simulink model "Desain_AMC"  (R2023a)
settings: Solver=VariableStepAuto  StartTime=0.0  StopTime=0.5  RelTol=1e-3
libraries: spsSeriesRLCBranchLib x18, dspstat3 x11, spsVoltageMeasurementLib x8, spsCurrentMeasurementLib x4, eePowerMeasurement x4, spsACVoltageSourceLib x2, spsDCVoltageSourceLib x2, spsRMSLib x1, sps_lib x1
settings Model: Creator=rne2p  LastModifiedBy=rne2p

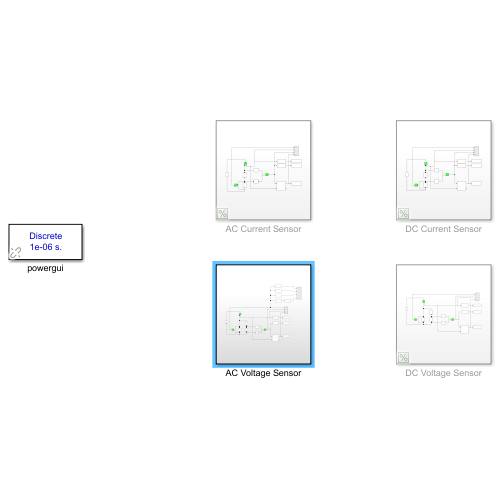
[thumbnail: Simulink's stored preview of the top-level diagram]
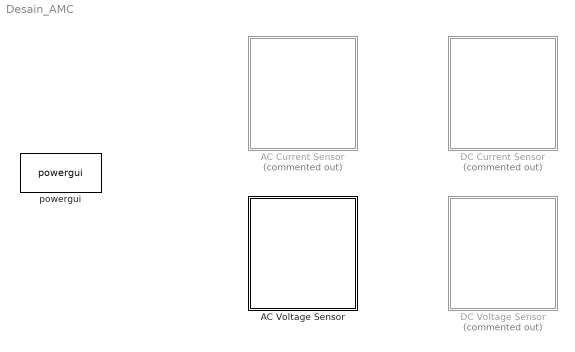
== system Desain_AMC ==
  AC Current Sensor : Subsystem  Commented=on
  AC Voltage Sensor : Subsystem
  DC Current Sensor : Subsystem  Commented=on
  DC Voltage Sensor : Subsystem  Commented=on
  powergui : sps_lib/powergui  Priority=1  SimulationMode=Discrete  SampleTime=1e-6  frequency=60  Iterations=50  frequencyindice=50  Pbase=100e6  ErrMax=1e-4  UnitsV=kV  UnitsW=MW  buscounter=0  FunctionMessages=off  echomessages=off  EnableUseOfTLC=off  CurrentSourceSwitches=off  DisableSnubberDevices=off  DisableRonSwitches=off  DisableVfSwitches=off  DisplayEquations=off  AutomaticDiscreteSolvers=off  SolverType=Tustin/Backward Euler (TBE)  Interpol=off  ExternalGateDelay=off  methode=off  Ts=100  x0status=blocks  SPID=on  SwTol=0  HookPort=off  NonlinearTolerance=1e-4  nMaxIteration=100  ContinueOnMaxIteration=off  RestoreLinks=warning  ResistiveCurrentMeasurement=off  Frange=[0:2:500]  Ylog=off  Xlog=on  ShowGrid=off  save=off  variable=ZData  structure=0  ZoomFFT=off  StartTime=0.0  cycles=1  DisplayStyle=1  fundamental=60  FreqAxis=off  MaxFrequency=1000  frequencyindicesteady=1  RmsSteady=1  display=off

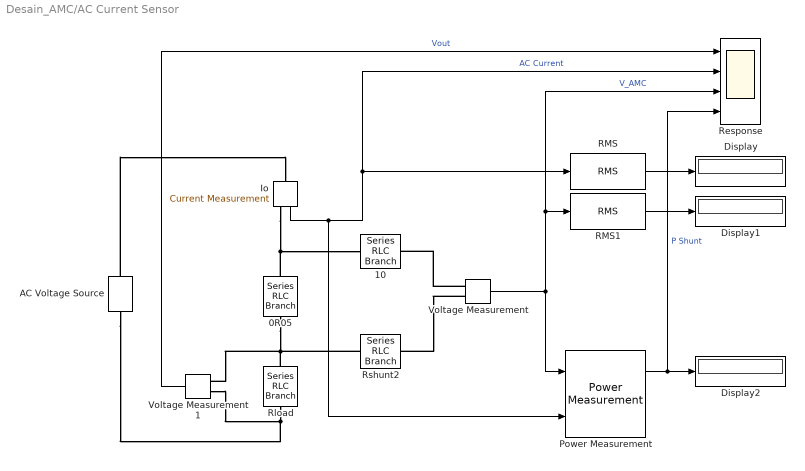
== system Desain_AMC/AC Current Sensor ==
  0R05 : spsSeriesRLCBranchLib/Series RLC Branch  LConnTagsString=__new0  RConnTagsString=__new0  BranchType=R  Resistance=50e-3  Inductance=100e-03  SetiL0=off  InitialCurrent=0  Capacitance=1.0  Setx0=off  InitialVoltage=0  Measurements=None
  10 : spsSeriesRLCBranchLib/Series RLC Branch  LConnTagsString=__new0  RConnTagsString=__new0  BranchType=R  Resistance=100  Inductance=100e-03  SetiL0=off  InitialCurrent=0  Capacitance=1.0  Setx0=off  InitialVoltage=0  Measurements=None
  AC Voltage Source : spsACVoltageSourceLib/AC Voltage Source  Amplitude=220*sqrt(2)  Phase=0  Frequency=50  SampleTime=0  Measurements=None  BusType=swing  Pref=10e3  Qref=0  Qmin=-inf  Qmax=+inf
  Display : Display
  Display1 : Display
  Display2 : Display
  Io : spsCurrentMeasurementLib/Current Measurement  Tag=PoWeRsYsTeMmEaSuReMeNt  PhasorSimulation=off  OutputType=Magnitude  PSBequivalent=0
      settings: AttributesFormatString=\n
  Power Measurement : eePowerMeasurement/Power Measurement  LabelModeActiveChoice=Continuous  F=50  K=1  Ts=0
  RMS : dspstat3/RMS  run=on  directionMode=Each column  dimension=1  InputProcessing=Columns as channels (frame based)  reset_popup=None
  RMS1 : dspstat3/RMS  run=on  directionMode=Each column  dimension=1  InputProcessing=Columns as channels (frame based)  reset_popup=None
  Response : Scope  NumInputPorts=4
  Rload : spsSeriesRLCBranchLib/Series RLC Branch  LConnTagsString=__new0  RConnTagsString=__new0  BranchType=R  Resistance=220/1  Inductance=100e-03  SetiL0=off  InitialCurrent=0  Capacitance=1.0  Setx0=off  InitialVoltage=0  Measurements=None
  Rshunt2 : spsSeriesRLCBranchLib/Series RLC Branch  LConnTagsString=__new0  RConnTagsString=__new0  BranchType=R  Resistance=100  Inductance=100e-03  SetiL0=off  InitialCurrent=0  Capacitance=1.0  Setx0=off  InitialVoltage=0  Measurements=None
  Voltage Measurement : spsVoltageMeasurementLib/Voltage Measurement  PhasorSimulation=off  OutputType=Complex  PSBequivalent=0
  Voltage Measurement1 : spsVoltageMeasurementLib/Voltage Measurement  PhasorSimulation=off  OutputType=Complex  PSBequivalent=0
  wires:
  Voltage Measurement1/1 -> Response/1  "Vout"
  Voltage Measurement/1 -> Power Measurement/1, Response/3, RMS1/1  "V_AMC"
  Io/1 -> Response/2, RMS/1, Power Measurement/2  "AC Current"
  RMS/1 -> Display/1
  Power Measurement/1 -> Response/4, Display2/1  "P Shunt"
  RMS1/1 -> Display1/1
  connections:
  Rload/RConn1 -- AC Voltage Source/LConn1 -- Voltage Measurement1/LConn2
  Voltage Measurement/LConn1 -- 10/RConn1
  0R05/LConn1 -- Io/RConn1 -- 10/LConn1
  Rload/LConn1 -- Rshunt2/LConn1 -- 0R05/RConn1 -- Voltage Measurement1/LConn1
  AC Voltage Source/RConn1 -- Io/LConn1
  Voltage Measurement/LConn2 -- Rshunt2/RConn1

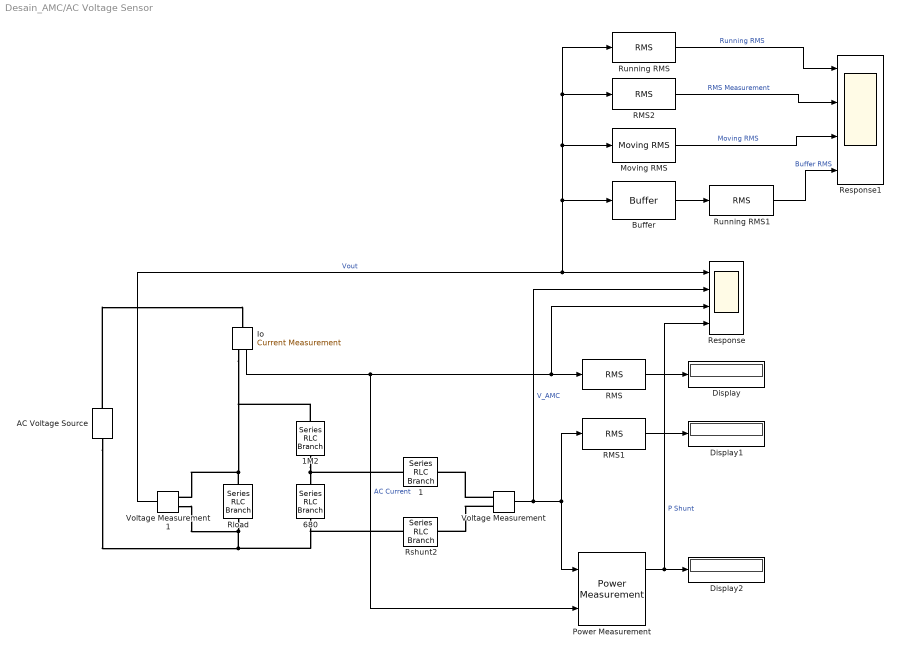
== system Desain_AMC/AC Voltage Sensor ==
  1 : spsSeriesRLCBranchLib/Series RLC Branch  LConnTagsString=__new0  RConnTagsString=__new0  BranchType=R  Resistance=10  Inductance=100e-03  SetiL0=off  InitialCurrent=0  Capacitance=1.0  Setx0=off  InitialVoltage=0  Measurements=None
  1M2 : spsSeriesRLCBranchLib/Series RLC Branch  LConnTagsString=__new0  RConnTagsString=__new0  BranchType=R  Resistance=1.2*10^6  Inductance=100e-03  SetiL0=off  InitialCurrent=0  Capacitance=1.0  Setx0=off  InitialVoltage=0  Measurements=None
  680 : spsSeriesRLCBranchLib/Series RLC Branch  LConnTagsString=__new0  RConnTagsString=__new0  BranchType=R  Resistance=680  Inductance=100e-03  SetiL0=off  InitialCurrent=0  Capacitance=1.0  Setx0=off  InitialVoltage=0  Measurements=None
  AC Voltage Source : spsACVoltageSourceLib/AC Voltage Source  Amplitude=220*sqrt(2)  Phase=0  Frequency=50  SampleTime=0  Measurements=None  BusType=swing  Pref=10e3  Qref=0  Qmin=-inf  Qmax=+inf
  Buffer : Buffer  N=200  OutputFrames=off
  Display : Display
  Display1 : Display
  Display2 : Display
  Io : spsCurrentMeasurementLib/Current Measurement  Tag=PoWeRsYsTeMmEaSuReMeNt  PhasorSimulation=off  OutputType=Magnitude  PSBequivalent=0
      settings: AttributesFormatString=\n
  Moving RMS : dspstat3/Moving RMS  Method=Sliding window  ForgettingFactorPort=off  SpecifyWindowLength=on  WindowLength=20000  OverlapLength=19999  AllowArbitraryInputLength=off  ForgettingFactor=0.9  SimulateUsing=Code generation
  Power Measurement : eePowerMeasurement/Power Measurement  LabelModeActiveChoice=Continuous  F=50  K=1  Ts=0
  RMS : dspstat3/RMS  run=on  directionMode=Each column  dimension=1  InputProcessing=Columns as channels (frame based)  reset_popup=None
  RMS1 : dspstat3/RMS  run=on  directionMode=Each column  dimension=1  InputProcessing=Columns as channels (frame based)  reset_popup=None
  RMS2 : spsRMSLib/RMS  TrueRMS=on  Freq=50  RMSInit=0  Ts=0
  Response : Scope  NumInputPorts=4
  Response1 : Scope  NumInputPorts=4
  Rload : spsSeriesRLCBranchLib/Series RLC Branch  LConnTagsString=__new0  RConnTagsString=__new0  BranchType=R  Resistance=220/2  Inductance=100e-03  SetiL0=off  InitialCurrent=0  Capacitance=1.0  Setx0=off  InitialVoltage=0  Measurements=None
  Rshunt2 : spsSeriesRLCBranchLib/Series RLC Branch  LConnTagsString=__new0  RConnTagsString=__new0  BranchType=R  Resistance=10  Inductance=100e-03  SetiL0=off  InitialCurrent=0  Capacitance=1.0  Setx0=off  InitialVoltage=0  Measurements=None
  Running RMS : dspstat3/RMS  run=on  directionMode=Each column  dimension=1  InputProcessing=Columns as channels (frame based)  reset_popup=None
  Running RMS1 : dspstat3/RMS  run=off  directionMode=Entire input  dimension=1  InputProcessing=Columns as channels (frame based)  reset_popup=None
  Voltage Measurement : spsVoltageMeasurementLib/Voltage Measurement  PhasorSimulation=off  OutputType=Complex  PSBequivalent=0
  Voltage Measurement1 : spsVoltageMeasurementLib/Voltage Measurement  PhasorSimulation=off  OutputType=Complex  PSBequivalent=0
  wires:
  RMS1/1 -> Display1/1
  Power Measurement/1 -> Response/4, Display2/1  "P Shunt"
  RMS/1 -> Display/1
  Io/1 -> Power Measurement/2, Response/3, RMS/1  "AC Current"
  Voltage Measurement/1 -> Response/2, RMS1/1, Power Measurement/1  "V_AMC"
  Voltage Measurement1/1 -> Buffer/1, RMS2/1, Running RMS/1, Moving RMS/1, Response/1  "Vout"
  Running RMS/1 -> Response1/1  "Running RMS"
  RMS2/1 -> Response1/2  "RMS Measurement"
  Moving RMS/1 -> Response1/3  "Moving RMS"
  Buffer/1 -> Running RMS1/1
  Running RMS1/1 -> Response1/4  "Buffer RMS"
  connections:
  Voltage Measurement/LConn2 -- Rshunt2/RConn1
  AC Voltage Source/RConn1 -- Io/LConn1
  Rload/LConn1 -- 1M2/LConn1 -- Io/RConn1 -- Voltage Measurement1/LConn1
  Voltage Measurement/LConn1 -- 1/RConn1
  Voltage Measurement1/LConn2 -- Rshunt2/LConn1 -- 680/RConn1 -- AC Voltage Source/LConn1 -- Rload/RConn1
  1M2/RConn1 -- 1/LConn1 -- 680/LConn1

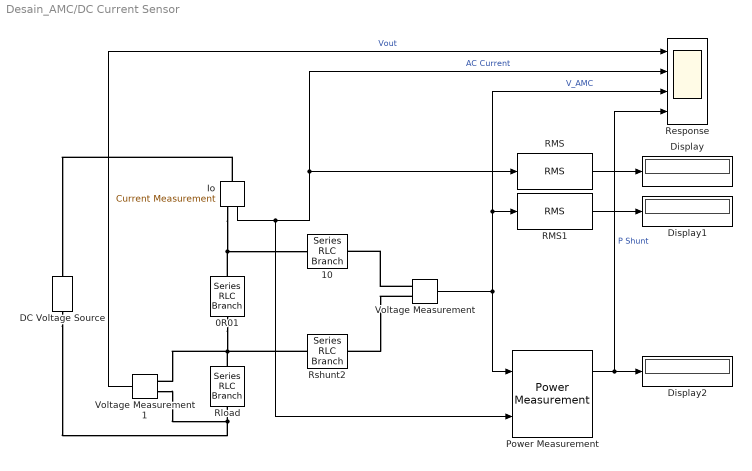
== system Desain_AMC/DC Current Sensor ==
  0R01 : spsSeriesRLCBranchLib/Series RLC Branch  LConnTagsString=__new0  RConnTagsString=__new0  BranchType=R  Resistance=10e-3  Inductance=100e-03  SetiL0=off  InitialCurrent=0  Capacitance=1.0  Setx0=off  InitialVoltage=0  Measurements=None
  10 : spsSeriesRLCBranchLib/Series RLC Branch  LConnTagsString=__new0  RConnTagsString=__new0  BranchType=R  Resistance=10  Inductance=100e-03  SetiL0=off  InitialCurrent=0  Capacitance=1.0  Setx0=off  InitialVoltage=0  Measurements=None
  DC Voltage Source : spsDCVoltageSourceLib/DC Voltage Source  Amplitude=24  Measurements=None
  Display : Display
  Display1 : Display
  Display2 : Display
  Io : spsCurrentMeasurementLib/Current Measurement  Tag=PoWeRsYsTeMmEaSuReMeNt  PhasorSimulation=off  OutputType=Magnitude  PSBequivalent=0
      settings: AttributesFormatString=\n
  Power Measurement : eePowerMeasurement/Power Measurement  LabelModeActiveChoice=Continuous  F=50  K=1  Ts=0
  RMS : dspstat3/RMS  run=on  directionMode=Each column  dimension=1  InputProcessing=Columns as channels (frame based)  reset_popup=None
  RMS1 : dspstat3/RMS  run=on  directionMode=Each column  dimension=1  InputProcessing=Columns as channels (frame based)  reset_popup=None
  Response : Scope  NumInputPorts=4
  Rload : spsSeriesRLCBranchLib/Series RLC Branch  LConnTagsString=__new0  RConnTagsString=__new0  BranchType=R  Resistance=24/25  Inductance=100e-03  SetiL0=off  InitialCurrent=0  Capacitance=1.0  Setx0=off  InitialVoltage=0  Measurements=None
  Rshunt2 : spsSeriesRLCBranchLib/Series RLC Branch  LConnTagsString=__new0  RConnTagsString=__new0  BranchType=R  Resistance=10  Inductance=100e-03  SetiL0=off  InitialCurrent=0  Capacitance=1.0  Setx0=off  InitialVoltage=0  Measurements=None
  Voltage Measurement : spsVoltageMeasurementLib/Voltage Measurement  PhasorSimulation=off  OutputType=Complex  PSBequivalent=0
  Voltage Measurement1 : spsVoltageMeasurementLib/Voltage Measurement  PhasorSimulation=off  OutputType=Complex  PSBequivalent=0
  wires:
  Voltage Measurement1/1 -> Response/1  "Vout"
  Voltage Measurement/1 -> Power Measurement/1, Response/3, RMS1/1  "V_AMC"
  Io/1 -> Response/2, RMS/1, Power Measurement/2  "AC Current"
  RMS/1 -> Display/1
  Power Measurement/1 -> Response/4, Display2/1  "P Shunt"
  RMS1/1 -> Display1/1
  connections:
  Voltage Measurement1/LConn2 -- DC Voltage Source/LConn1 -- Rload/RConn1
  Voltage Measurement/LConn1 -- 10/RConn1
  0R01/LConn1 -- Io/RConn1 -- 10/LConn1
  Rload/LConn1 -- Rshunt2/LConn1 -- 0R01/RConn1 -- Voltage Measurement1/LConn1
  Voltage Measurement/LConn2 -- Rshunt2/RConn1
  Io/LConn1 -- DC Voltage Source/RConn1

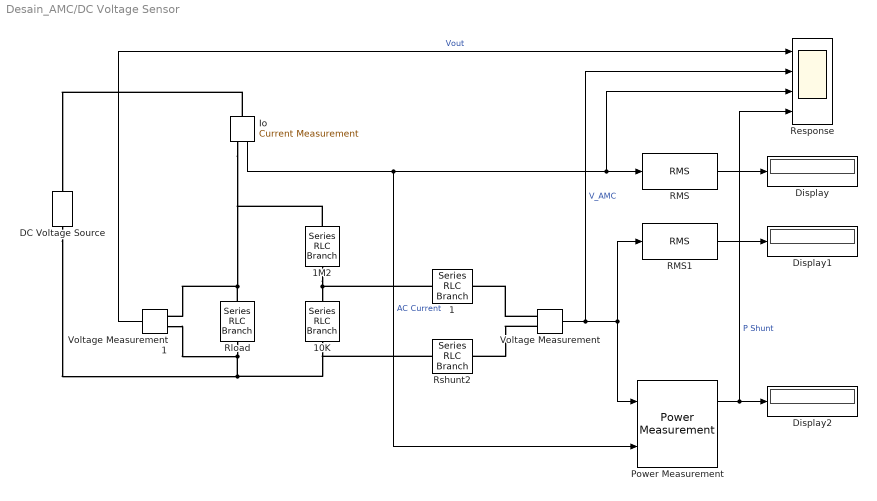
== system Desain_AMC/DC Voltage Sensor ==
  1 : spsSeriesRLCBranchLib/Series RLC Branch  LConnTagsString=__new0  RConnTagsString=__new0  BranchType=R  Resistance=10  Inductance=100e-03  SetiL0=off  InitialCurrent=0  Capacitance=1.0  Setx0=off  InitialVoltage=0  Measurements=None
  10K : spsSeriesRLCBranchLib/Series RLC Branch  LConnTagsString=__new0  RConnTagsString=__new0  BranchType=R  Resistance=10000  Inductance=100e-03  SetiL0=off  InitialCurrent=0  Capacitance=1.0  Setx0=off  InitialVoltage=0  Measurements=None
  1M2 : spsSeriesRLCBranchLib/Series RLC Branch  LConnTagsString=__new0  RConnTagsString=__new0  BranchType=R  Resistance=1.2*10^6  Inductance=100e-03  SetiL0=off  InitialCurrent=0  Capacitance=1.0  Setx0=off  InitialVoltage=0  Measurements=None
  DC Voltage Source : spsDCVoltageSourceLib/DC Voltage Source  Amplitude=24  Measurements=None
  Display : Display
  Display1 : Display
  Display2 : Display
  Io : spsCurrentMeasurementLib/Current Measurement  Tag=PoWeRsYsTeMmEaSuReMeNt  PhasorSimulation=off  OutputType=Magnitude  PSBequivalent=0
      settings: AttributesFormatString=\n
  Power Measurement : eePowerMeasurement/Power Measurement  LabelModeActiveChoice=Continuous  F=50  K=1  Ts=0
  RMS : dspstat3/RMS  run=on  directionMode=Each column  dimension=1  InputProcessing=Columns as channels (frame based)  reset_popup=None
  RMS1 : dspstat3/RMS  run=on  directionMode=Each column  dimension=1  InputProcessing=Columns as channels (frame based)  reset_popup=None
  Response : Scope  NumInputPorts=4
  Rload : spsSeriesRLCBranchLib/Series RLC Branch  LConnTagsString=__new0  RConnTagsString=__new0  BranchType=R  Resistance=24/1  Inductance=100e-03  SetiL0=off  InitialCurrent=0  Capacitance=1.0  Setx0=off  InitialVoltage=0  Measurements=None
  Rshunt2 : spsSeriesRLCBranchLib/Series RLC Branch  LConnTagsString=__new0  RConnTagsString=__new0  BranchType=R  Resistance=10  Inductance=100e-03  SetiL0=off  InitialCurrent=0  Capacitance=1.0  Setx0=off  InitialVoltage=0  Measurements=None
  Voltage Measurement : spsVoltageMeasurementLib/Voltage Measurement  PhasorSimulation=off  OutputType=Complex  PSBequivalent=0
  Voltage Measurement1 : spsVoltageMeasurementLib/Voltage Measurement  PhasorSimulation=off  OutputType=Complex  PSBequivalent=0
  wires:
  RMS1/1 -> Display1/1
  Power Measurement/1 -> Response/4, Display2/1  "P Shunt"
  RMS/1 -> Display/1
  Io/1 -> Power Measurement/2, Response/3, RMS/1  "AC Current"
  Voltage Measurement/1 -> Response/2, RMS1/1, Power Measurement/1  "V_AMC"
  Voltage Measurement1/1 -> Response/1  "Vout"
  connections:
  Voltage Measurement/LConn2 -- Rshunt2/RConn1
  Rload/LConn1 -- 1M2/LConn1 -- Io/RConn1 -- Voltage Measurement1/LConn1
  Voltage Measurement/LConn1 -- 1/RConn1
  Voltage Measurement1/LConn2 -- DC Voltage Source/LConn1 -- Rshunt2/LConn1 -- 10K/RConn1 -- Rload/RConn1
  1M2/RConn1 -- 1/LConn1 -- 10K/LConn1
  Io/LConn1 -- DC Voltage Source/RConn1
